simulink model "Sistema_radar"  (R2015a)
settings: Solver=ode45  StartTime=0.0  StopTime=200  FixedStep=.03  RelTol=1e-3
libraries: canmsglib x4, simulink x1
settings Model: Creator=vmaraccini  LastModifiedBy=Administrator

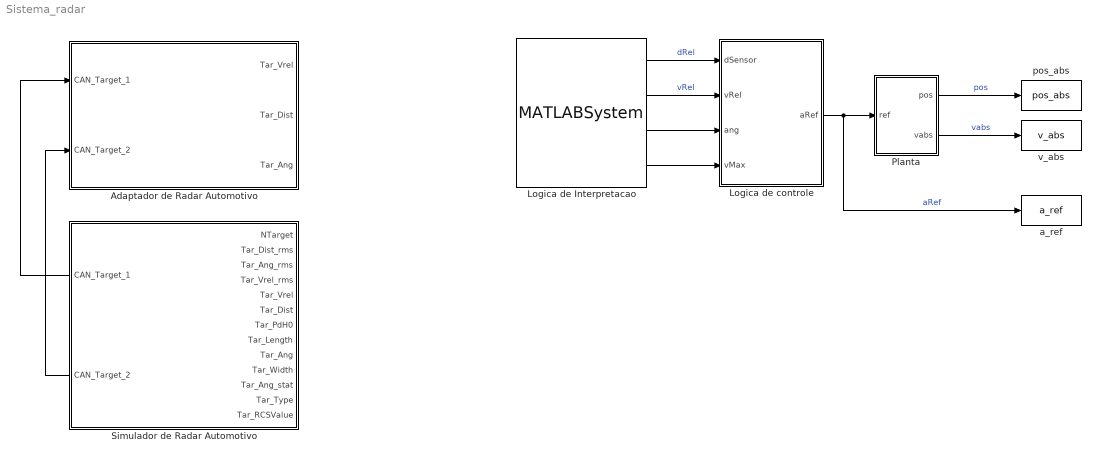
== system Sistema_radar ==
  Adaptador de Radar Automotivo : Subsystem
  Logica de Interpretacao : MATLABSystem  System=Interpretacao  SimulateUsing=Interpreted execution
      mask Type: Interpretacao
      mask Display:
      | disp('Interpretacao');
      | port_label('input',1,'vrel');
      | port_label('input',2,'dist');
      | port_label('input',3,'ang');
      | port_label('output',1,'d');
      | port_label('output',2,'v');
      | port_label('output',3,'a');
      | port_label('output',4,'max');
  Logica de controle : Subsystem
  Planta : Subsystem
  Simulador de Radar Automotivo : Subsystem
  a_ref : ToWorkspace  VariableName=a_ref  SaveFormat=Timeseries  SampleTime=-1
  pos_abs : ToWorkspace  VariableName=pos_abs  SaveFormat=Timeseries  SampleTime=-1
  v_abs : ToWorkspace  VariableName=v_abs  SaveFormat=Timeseries  SampleTime=-1
  wires:
  Planta/2(vabs) -> v_abs/1  "vabs"
  Logica de controle/1(aRef) -> a_ref/1, Planta/1(ref)  "aRef"
  Planta/1(pos) -> pos_abs/1  "pos"
  Simulador de Radar Automotivo/1(CAN_Target_1) -> Adaptador de Radar Automotivo/1(CAN_Target_1)
  Simulador de Radar Automotivo/2(CAN_Target_2) -> Adaptador de Radar Automotivo/2(CAN_Target_2)
  Logica de Interpretacao/1 -> Logica de controle/1(dSensor)  "dRel"
  Logica de Interpretacao/2 -> Logica de controle/2(vRel)  "vRel"
  Logica de Interpretacao/4 -> Logica de controle/4(vMax)
  Logica de Interpretacao/3 -> Logica de controle/3(ang)

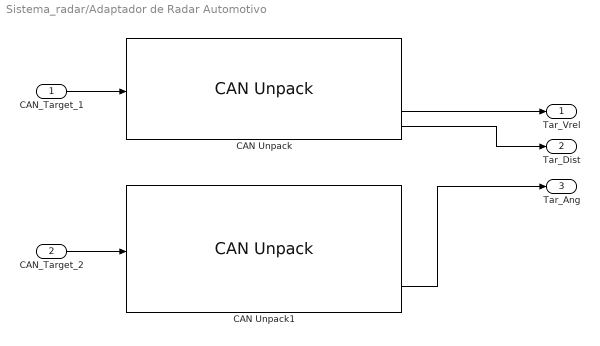
== system Sistema_radar/Adaptador de Radar Automotivo ==
  CAN_Target_1 : Inport
  CAN_Target_2 : Inport  Port=2
  CAN Unpack : canmsglib/CAN Unpack  MsgList=(none)  MsgName=CAN1_Target_1  MsgIDType=Standard (11-bit identifier)  MsgIdentifier=1793  MsgLength=8  SignalInfo=NoOfTarget_1$0$8$2$2$1$0$1$0$-Inf$Inf$#Tar_Dist_rms$8$8$2$2$1$0$0.1$-10$-Inf$Inf$#Tar_Ang_rms$17$7$2$2$1$0$0.1$0$-Inf$Inf$#Tar_Vrel_rms$24$9$2$2$1$0$0.03$-5$-Inf$Inf$#Tar_Vrel$44$12$2$2$1$0$0.03$-25$-Inf$Inf$#Tar_Dist$48$11$2$1$1$0$0.1$0$-Inf$Inf$#  NSignals=6  IDPort=off  TimestampPort=off  ErrorPort=off  RemotePort=off  LengthPort=off  StatusPort=off  StartBits=str2num('[int32(0);int32(8);int32(17);int32(24);int32(44);int32(48)]')  SignalSizes=str2num('[int32(8);int32(8);int32(7);int32(9);int32(12);int32(11)]')  ByteOrders=str2num('[int32(2);int32(2);int32(2);int32(2);int32(2);int32(2)]')  DataTypes=str2num('[int32(2);int32(2);int32(2);int32(2);int32(2);int32(1)]')  MultiplexTypes=str2num('[int32(1);int32(1);int32(1);int32(1);int32(1);int32(1)]')  MultiplexValues=str2num('[double(0);double(0);double(0);double(0);double(0);double(0)]')  Factors=str2num('[double(1);double(0.1);double(0.1);double(0.03);double(0.03);double(0.1)]')  Offsets=str2num('[double(0);double(-10);double(0);double(-5);double(-25);double(0)]')  Minimums=str2num('[double(-Inf);double(-Inf);double(-Inf);double(-Inf);double(-Inf);double(-Inf)]')  Maximums=str2num('[double(Inf);double(Inf);double(Inf);double(Inf);double(Inf);double(Inf)]')
  CAN Unpack1 : canmsglib/CAN Unpack  MsgList=(none)  MsgName=CAN1_Target_2  MsgIDType=Standard (11-bit identifier)  MsgIdentifier=1794  MsgLength=8  SignalInfo=NoOfTarget_2$0$8$2$2$1$0$1$0$-Inf$Inf$#Tar_PdH0$9$7$2$2$1$0$0.01$0$-Inf$Inf$#Tar_Length$16$9$2$2$1$0$0.1$0$-Inf$Inf$#Tar_Width$32$9$2$2$1$0$0.1$0$-Inf$Inf$#Tar_Ang_stat$44$2$2$2$1$0$1$0$-Inf$Inf$#Tar_Type$46$2$2$2$1$0$1$0$-Inf$Inf$#Tar_Ang$50$10$2$2$1$0$0.1$-30$-Inf$Inf$#Tar_RCSValue$56$10$2$2$1$0$0.1$-50$-Inf$Inf$#  NSignals=8  IDPort=off  TimestampPort=off  ErrorPort=off  RemotePort=off  LengthPort=off  StatusPort=off  StartBits=str2num('[int32(0);int32(9);int32(16);int32(32);int32(44);int32(46);int32(50);int32(56)]')  SignalSizes=str2num('[int32(8);int32(7);int32(9);int32(9);int32(2);int32(2);int32(10);int32(10)]')  ByteOrders=str2num('[int32(2);int32(2);int32(2);int32(2);int32(2);int32(2);int32(2);int32(2)]')  DataTypes=str2num('[int32(2);int32(2);int32(2);int32(2);int32(2);int32(2);int32(2);int32(2)]')  MultiplexTypes=str2num('[int32(1);int32(1);int32(1);int32(1);int32(1);int32(1);int32(1);int32(1)]')  MultiplexValues=str2num('[double(0);double(0);double(0);double(0);double(0);double(0);double(0);double(0)]')  Factors=str2num('[double(1);double(0.01);double(0.1);double(0.1);double(1);double(1);double(0.1);double(0.1)]')  Offsets=str2num('[double(0);double(0);double(0);double(0);double(0);double(0);double(-30);double(-50)]')  Minimums=str2num('[double(-Inf);double(-Inf);double(-Inf);double(-Inf);double(-Inf);double(-Inf);double(-Inf);double(-Inf)]')  Maximums=str2num('[double(Inf);double(Inf);double(Inf);double(Inf);double(Inf);double(Inf);double(Inf);double(Inf)]')
  Tar_Vrel : Outport
  Tar_Dist : Outport  Port=2
  Tar_Ang : Outport  Port=3
  wires:
  CAN Unpack/6 -> Tar_Dist/1
  CAN Unpack1/7 -> Tar_Ang/1
  CAN Unpack/5 -> Tar_Vrel/1
  CAN_Target_2/1 -> CAN Unpack1/1
  CAN_Target_1/1 -> CAN Unpack/1

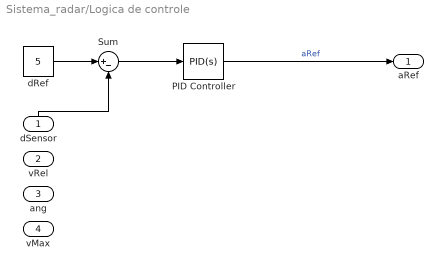
== system Sistema_radar/Logica de controle ==
  dSensor : Inport
  vRel : Inport  Port=2
  ang : Inport  Port=3
  vMax : Inport  Port=4
  PID Controller : simulink/Continuous/PID Controller  Controller=PID  TimeDomain=Continuous-time  SampleTime=-1  IntegratorMethod=Forward Euler  FilterMethod=Forward Euler  Form=Parallel  UseFilter=on  ControllerParametersSource=internal  P=1  I=0  D=2  N=100  InitialConditionSource=internal  InitialConditionForIntegrator=0  InitialConditionForFilter=0  ExternalReset=none  LimitOutput=off  UpperSaturationLimit=inf  LowerSaturationLimit=-inf  LinearizeAsGain=on  AntiWindupMode=none  Kb=1  TrackingMode=off  Kt=1  PParamMin=[]  PParamMax=[]  IParamMin=[]  IParamMax=[]  DParamMin=[]  DParamMax=[]  NParamMin=[]  NParamMax=[]  KbParamMin=[]  KbParamMax=[]  KtParamMin=[]  KtParamMax=[]  POutMin=[]  POutMax=[]  IOutMin=[]  IOutMax=[]  DOutMin=[]  DOutMax=[]  NOutMin=[]  NOutMax=[]  KbOutMin=[]  KbOutMax=[]  KtOutMin=[]  KtOutMax=[]  IntegratorOutMin=[]  IntegratorOutMax=[]  FilterOutMin=[]  FilterOutMax=[]  SumOutMin=[]  SumOutMax=[]  SumI1OutMin=[]  SumI1OutMax=[]  SumI2OutMin=[]  SumI2OutMax=[]  SumI3OutMin=[]  SumI3OutMax=[]  SumDOutMin=[]  SumDOutMax=[]  SaturationOutMin=[]  SaturationOutMax=[]  IntegratorContinuousStateAttributes=''  IntegratorStateMustResolveToSignalObject=off  IntegratorRTWStateStorageClass=Auto  FilterContinuousStateAttributes=''  FilterStateMustResolveToSignalObject=off  FilterRTWStateStorageClass=Auto  DifferentiatorICPrevScaledInput=0  DifferentiatorOutMin=[]  DifferentiatorOutMax=[]
  Sum : Sum  Inputs=|+-
  dRef : Constant  Value=5
  aRef : Outport
  wires:
  dSensor/1 -> Sum/2
  Sum/1 -> PID Controller/1
  dRef/1 -> Sum/1
  PID Controller/1 -> aRef/1  "aRef"

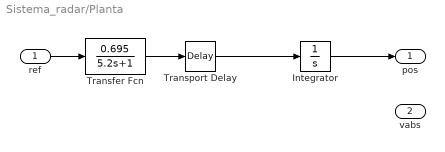
== system Sistema_radar/Planta ==
  ref : Inport
  Integrator : Integrator
  Transfer Fcn : TransferFcn  Numerator=[0 0.695]  Denominator=[5.2 1]
  Transport Delay : TransportDelay  DelayTime=0.5  InitialOutput=13.9
  pos : Outport
  vabs : Outport  Port=2
  wires:
  Integrator/1 -> pos/1
  Transfer Fcn/1 -> Transport Delay/1
  ref/1 -> Transfer Fcn/1
  Transport Delay/1 -> Integrator/1

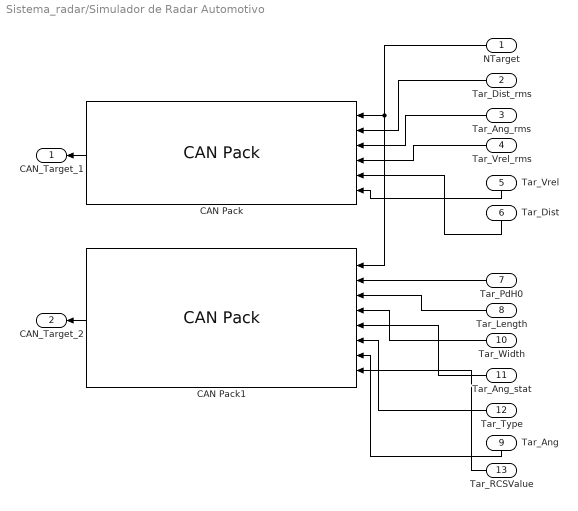
== system Sistema_radar/Simulador de Radar Automotivo ==
  NTarget : Inport
  Tar_Dist_rms : Inport  Port=2
  Tar_Ang_rms : Inport  Port=3
  Tar_Vrel_rms : Inport  Port=4
  Tar_Vrel : Inport  Port=5
  Tar_Dist : Inport  Port=6
  Tar_PdH0 : Inport  Port=7
  Tar_Length : Inport  Port=8
  Tar_Ang : Inport  Port=9
  Tar_Width : Inport  Port=10
  Tar_Ang_stat : Inport  Port=11
  Tar_Type : Inport  Port=12
  Tar_RCSValue : Inport  Port=13
  CAN Pack : canmsglib/CAN Pack  MsgList=(none)  MsgName=CAN1_Target_1  MsgIDType=Standard (11-bit identifier)  MsgIdentifier=1793  MsgLength=8  SignalInfo=NoOfTarget_1$0$8$2$2$1$0$1$0$-Inf$Inf$#Tar_Dist_rms$8$8$2$2$1$0$0.1$-10$-Inf$Inf$#Tar_Ang_rms$17$7$2$2$1$0$0.1$0$-Inf$Inf$#Tar_Vrel_rms$24$9$2$2$1$0$0.03$-5$-Inf$Inf$#Tar_Vrel$44$12$2$2$1$0$0.03$-25$-Inf$Inf$#Tar_Dist$48$11$2$2$1$0$0.1$0$-Inf$Inf$#  NSignals=6  StartBits=str2num('[int32(0);int32(8);int32(17);int32(24);int32(44);int32(48)]')  SignalSizes=str2num('[int32(8);int32(8);int32(7);int32(9);int32(12);int32(11)]')  ByteOrders=str2num('[int32(2);int32(2);int32(2);int32(2);int32(2);int32(2)]')  DataTypes=str2num('[int32(2);int32(2);int32(2);int32(2);int32(2);int32(2)]')  MultiplexTypes=str2num('[int32(1);int32(1);int32(1);int32(1);int32(1);int32(1)]')  MultiplexValues=str2num('[double(0);double(0);double(0);double(0);double(0);double(0)]')  Factors=str2num('[double(1);double(0.1);double(0.1);double(0.03);double(0.03);double(0.1)]')  Offsets=str2num('[double(0);double(-10);double(0);double(-5);double(-25);double(0)]')  Minimums=str2num('[double(-Inf);double(-Inf);double(-Inf);double(-Inf);double(-Inf);double(-Inf)]')  Maximums=str2num('[double(Inf);double(Inf);double(Inf);double(Inf);double(Inf);double(Inf)]')  Remote=off
      settings: DataFormat=manually specified signals
  CAN Pack1 : canmsglib/CAN Pack  MsgList=(none)  MsgName=CAN1_Target_2  MsgIDType=Standard (11-bit identifier)  MsgIdentifier=1794  MsgLength=8  SignalInfo=NoOfTarget_2$0$8$2$2$1$0$1$0$-Inf$Inf$#Tar_PdH0$9$7$2$2$1$0$0.01$-10$-Inf$Inf$#Tar_Length$16$9$2$2$1$0$0.1$0$-Inf$Inf$#Tar_Width$32$9$2$2$1$0$.01$0$-Inf$Inf$#Tar_Ang_stat$44$2$2$2$1$0$1$0$-Inf$Inf$#Tar_Type$46$2$2$2$1$0$1$0$-Inf$Inf$#Tar_Ang$50$10$2$2$1$0$0.1$-30$-Inf$Inf$#Tar_RCSValue$56$10$2$2$1$0$0.1$-50$-Inf$Inf$#  NSignals=8  StartBits=str2num('[int32(0);int32(9);int32(16);int32(32);int32(44);int32(46);int32(50);int32(56)]')  SignalSizes=str2num('[int32(8);int32(7);int32(9);int32(9);int32(2);int32(2);int32(10);int32(10)]')  ByteOrders=str2num('[int32(2);int32(2);int32(2);int32(2);int32(2);int32(2);int32(2);int32(2)]')  DataTypes=str2num('[int32(2);int32(2);int32(2);int32(2);int32(2);int32(2);int32(2);int32(2)]')  MultiplexTypes=str2num('[int32(1);int32(1);int32(1);int32(1);int32(1);int32(1);int32(1);int32(1)]')  MultiplexValues=str2num('[double(0);double(0);double(0);double(0);double(0);double(0);double(0);double(0)]')  Factors=str2num('[double(1);double(0.01);double(0.1);double(.01);double(1);double(1);double(0.1);double(0.1)]')  Offsets=str2num('[double(0);double(-10);double(0);double(0);double(0);double(0);double(-30);double(-50)]')  Minimums=str2num('[double(-Inf);double(-Inf);double(-Inf);double(-Inf);double(-Inf);double(-Inf);double(-Inf);double(-Inf)]')  Maximums=str2num('[double(Inf);double(Inf);double(Inf);double(Inf);double(Inf);double(Inf);double(Inf);double(Inf)]')  Remote=off
      settings: DataFormat=manually specified signals
  CAN_Target_1 : Outport
  CAN_Target_2 : Outport  Port=2
  wires:
  CAN Pack/1 -> CAN_Target_1/1
  CAN Pack1/1 -> CAN_Target_2/1
  Tar_Vrel_rms/1 -> CAN Pack/4
  Tar_Width/1 -> CAN Pack1/4
  NTarget/1 -> CAN Pack1/1, CAN Pack/1
  Tar_Ang_stat/1 -> CAN Pack1/5
  Tar_Dist_rms/1 -> CAN Pack/2
  Tar_PdH0/1 -> CAN Pack1/2
  Tar_Dist/1 -> CAN Pack/5
  Tar_Ang_rms/1 -> CAN Pack/3
  Tar_Length/1 -> CAN Pack1/3
  Tar_RCSValue/1 -> CAN Pack1/8
  Tar_Ang/1 -> CAN Pack1/7
  Tar_Vrel/1 -> CAN Pack/6
  Tar_Type/1 -> CAN Pack1/6
